simulink model "test_sim"  (Simulink 10.3)
settings: Solver=ode1  StartTime=0.0  StopTime=5  FixedStep=0.001  RelTol=1e-3  EnableMultiTasking=on
settings Model: Creator=ljk  LastModifiedBy=fu  ExtModeTrigMode=oneshot  ExtModeArmWhenConnect=off
settings OptimizationCC: BlockReduction=off  BooleanDataType=off
settings DebuggingCC: SaveWithParameterizedLinksMsg=none  SignalResolutionControl=TryResolveAllWithWarning  MultiTaskDSMMsg=warning  MultiTaskCondExecSysMsg=none
settings HardwareCC: TargetUnknown=on

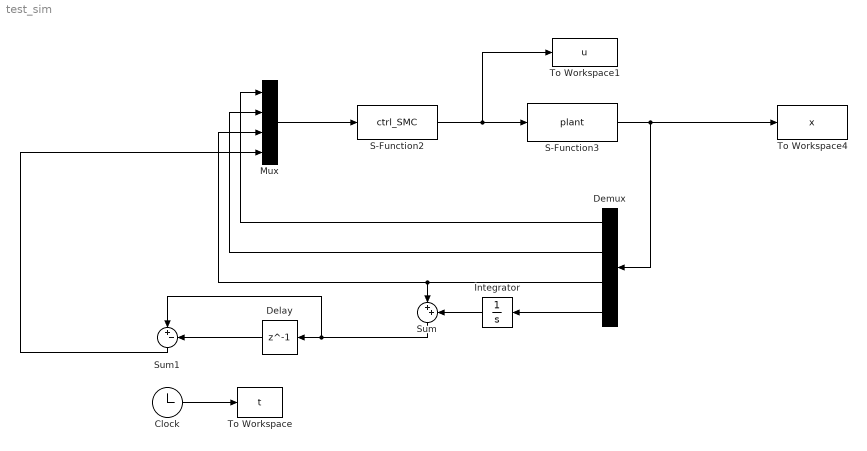
== system test_sim ==
  Clock : Clock
  Delay : Delay  DelayLength=1  InitialCondition=0
  Demux : Demux
  Integrator : Integrator
  Mux : Mux
  S-Function2 : S-Function  FunctionName=ctrl_SMC  SFunctionDeploymentMode=off  EnableBusSupport=off
  S-Function3 : S-Function  FunctionName=plant  SFunctionDeploymentMode=off  EnableBusSupport=off
  Sum : Sum  Inputs=|++
  Sum1 : Sum  Inputs=|+-
  To Workspace : ToWorkspace  VariableName=t  SampleTime=-1
  To Workspace1 : ToWorkspace  VariableName=u  SampleTime=-1
  To Workspace4 : ToWorkspace  VariableName=x  SampleTime=-1
  wires:
  Clock/1 -> To Workspace/1
  S-Function3/1 -> Demux/1, To Workspace4/1
  S-Function2/1 -> S-Function3/1, To Workspace1/1
  Mux/1 -> S-Function2/1
  Integrator/1 -> Sum/2
  Sum/1 -> Sum1/1, Delay/1
  Delay/1 -> Sum1/2
  Demux/1 -> Mux/1
  Demux/4 -> Integrator/1
  Demux/3 -> Mux/3, Sum/1
  Sum1/1 -> Mux/4
  Demux/2 -> Mux/2
